simulink model "Model12"  (R2020a)
settings: Solver=ode15s  StartTime=0.0  StopTime=200  RelTol=1e-3
values from neighbouring files (symbols this model uses):
  Cf = 100000    [Model12_MATscript.m]
  Cr = 110000    [Model12_MATscript.m]
undefined symbols (not defined in the file or in its folder): a, a0, a1, a10, a11, a12, a13, a14, a15, a16, a17, a2, a3, a4, a5, a6, a7, a8, a9, alpha, Area, b, b1, b11, b12, b2, banking_indy, bankingON, C_fuel, camber, curveCenters, Cx, Cz, distanceThreshold, g, init_vel, init_x_pos, init_y_pos, init_yaw, IT, K_wear, l_f, l_r, longStraight, lookahead, m_fuel, mT, overlapThreshold, radius_second_lane, rho_0, rho_1, shortStraight, slipstreamON, trajec, turn, TyreContactAreaFront, TyreContactAreaRear, w1, w2
libraries: simulink x6
(part 2 of 2)

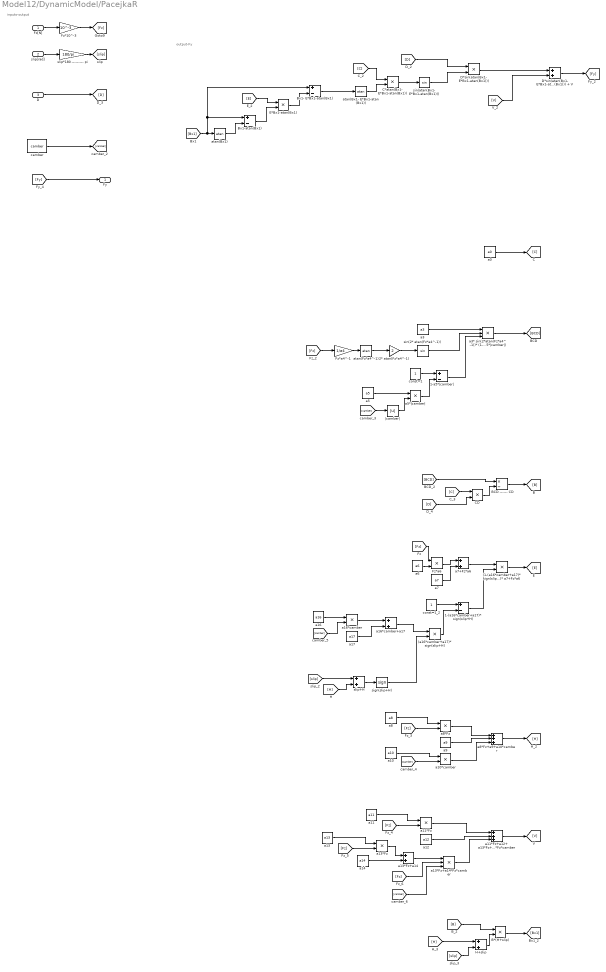
== system Model12/DynamicModel/PacejkaR ==
  note: inputs-output
  note: output-Fy
  Fz[N] : Inport  Unit=N
  slip[rad] : Inport  Port=2  Unit=rad
  D : Inport  Port=3
  (1-(a16*camber+a17)* sign(slip+H))* a7+Fz*a6 : Product
  (a16*camber+a17)* sign(slip+H) : Product
  1-(a16*camber+a17)* sign(slip+H) : Sum  Inputs=+-
  1-a5*|camber| : Sum  Inputs=+-
  2* atan(Fz*a4^-1) : Gain  Gain=2
  B*(H+slip) : Product
  BCD ------ CD : Product  Inputs=*/
  Bx1- E*Bx1-atan(Bx1) : Sum  Inputs=+-
  Bx1-atan(Bx1) : Sum  Inputs=+-
  C*atan(Bx1- E*Bx1-atan(Bx1)) : Product
  CD : Product
  D*sin(atan(Bx1- E*Bx1-atan(Bx1))) : Product
  D*sin(atan(Bx1- E*Bx1-atan(Bx1))) + V : Sum
  E*Bx1-atan(Bx1) : Product
  Fz*10^-3 : Gain  Gain=10^-3
  Fz*a4^-1 : Gain  Gain=1/a4
  Fz*a6 : Product
  H+slip : Sum
  a0 : Constant  Value=a0
  a10 : Constant  Value=a10
  a10*camber : Product
  a11 : Constant  Value=a11
  a11*Fz : Product
  a11*Fz+a12+ a13*Fz+a14*Fz*camber : Sum  Inputs=+++
  a12 : Constant  Value=a12
  a13 : Constant  Value=a13
  a13*Fz : Product
  a13*Fz+a14 : Sum
  a13*Fz+a14*Fz*camber : Product  Inputs=3
  a14 : Constant  Value=a14
  a16 : Constant  Value=a16
  a16*camber : Product
  a16*camber+a17 : Sum
  a17 : Constant  Value=a17
  a3 : Constant  Value=a3
  a3* sin(2*atan(Fz*a4^-1))* (1-a5*|camber|) : Product  Inputs=3
  a5 : Constant  Value=a5
  a5*|camber| : Product
  a6 : Constant  Value=a6
  a7 : Constant  Value=a7
  a7+Fz*a6 : Sum
  a8 : Constant  Value=a8
  a8*Fz : Product
  a8*Fz+a9+a10*camber : Sum  Inputs=+++
  a9 : Constant  Value=a9
  atan(Bx1) : Trigonometry  Operator=atan
  atan(Bx1- E*Bx1-atan(Bx1)) : Trigonometry  Operator=atan
  atan(Fz*a4^-1) : Trigonometry  Operator=atan
  camber : Constant  Value=camber
  const=1 : Constant
  const=1_2 : Constant
  sign(slip+H) : Signum  ZeroCross=off
  sin(2* atan(Fz*a4^-1)) : Trigonometry
  sin(atan(Bx1- E*Bx1-atan(Bx1))) : Trigonometry
  slip*180 --------- pi : Gain  Gain=180/pi
  slip+H : Sum
  |camber| : Abs
  Fy : Outport  Unit=N
  wires:
  C*atan(Bx1- E*Bx1-atan(Bx1))/1 -> sin(atan(Bx1- E*Bx1-atan(Bx1)))/1
  E*Bx1-atan(Bx1)/1 -> Bx1- E*Bx1-atan(Bx1)/2
  slip[rad]/1 -> slip*180 --------- pi/1
  1-a5*|camber|/1 -> a3* sin(2*atan(Fz*a4^-1))* (1-a5*|camber|)/3
  a10*camber/1 -> a8*Fz+a9+a10*camber/3
  |camber|/1 -> a5*|camber|/2
  a8/1 -> a8*Fz/1
  Fz*10^-3/1 -> [Fz]
  a0/1 -> [C]
  atan(Bx1- E*Bx1-atan(Bx1))/1 -> C*atan(Bx1- E*Bx1-atan(Bx1))/2
  [Fy] -> Fy/1
  Fz*a4^-1/1 -> atan(Fz*a4^-1)/1
  [B] -> B*(H+slip)/1
  [Fz] -> a8*Fz/2
  [Bx1] -> atan(Bx1)/1, Bx1-atan(Bx1)/1, Bx1- E*Bx1-atan(Bx1)/1
  [Fz] -> a13*Fz+a14*Fz*camber/2
  slip*180 --------- pi/1 -> [slip]
  2* atan(Fz*a4^-1)/1 -> sin(2* atan(Fz*a4^-1))/1
  [Fz] -> Fz*a6/1
  [slip] -> H+slip/2
  a11*Fz+a12+ a13*Fz+a14*Fz*camber/1 -> [V]
  a7+Fz*a6/1 -> (1-(a16*camber+a17)* sign(slip+H))* a7+Fz*a6/1
  [D] -> D*sin(atan(Bx1- E*Bx1-atan(Bx1)))/1
  a8*Fz+a9+a10*camber/1 -> [H]
  1-(a16*camber+a17)* sign(slip+H)/1 -> (1-(a16*camber+a17)* sign(slip+H))* a7+Fz*a6/2
  Bx1- E*Bx1-atan(Bx1)/1 -> atan(Bx1- E*Bx1-atan(Bx1))/1
  a3/1 -> a3* sin(2*atan(Fz*a4^-1))* (1-a5*|camber|)/1
  [camber] -> a16*camber/2
  [V] -> D*sin(atan(Bx1- E*Bx1-atan(Bx1))) + V/2
  [C] -> C*atan(Bx1- E*Bx1-atan(Bx1))/1
  B*(H+slip)/1 -> [Bx1]
  Fz[N]/1 -> Fz*10^-3/1
  camber/1 -> [camber]
  a11*Fz/1 -> a11*Fz+a12+ a13*Fz+a14*Fz*camber/1
  const=1/1 -> 1-a5*|camber|/1
  [Fz] -> a13*Fz/2
  a8*Fz/1 -> a8*Fz+a9+a10*camber/1
  [BCD] -> BCD ------ CD/1
  a14/1 -> a13*Fz+a14/2
  sin(atan(Bx1- E*Bx1-atan(Bx1)))/1 -> D*sin(atan(Bx1- E*Bx1-atan(Bx1)))/2
  sign(slip+H)/1 -> (a16*camber+a17)* sign(slip+H)/2
  a3* sin(2*atan(Fz*a4^-1))* (1-a5*|camber|)/1 -> [BCD]
  [camber] -> |camber|/1
  a13*Fz+a14/1 -> a13*Fz+a14*Fz*camber/1
  a9/1 -> a8*Fz+a9+a10*camber/2
  a16*camber/1 -> a16*camber+a17/1
  a12/1 -> a11*Fz+a12+ a13*Fz+a14*Fz*camber/2
  (1-(a16*camber+a17)* sign(slip+H))* a7+Fz*a6/1 -> [E]
  [Fz] -> Fz*a4^-1/1
  D*sin(atan(Bx1- E*Bx1-atan(Bx1))) + V/1 -> [Fy]
  BCD ------ CD/1 -> [B]
  a10/1 -> a10*camber/1
  [H] -> H+slip/1
  atan(Fz*a4^-1)/1 -> 2* atan(Fz*a4^-1)/1
  a16*camber+a17/1 -> (a16*camber+a17)* sign(slip+H)/1
  a11/1 -> a11*Fz/1
  a13*Fz/1 -> a13*Fz+a14/1
  a13*Fz+a14*Fz*camber/1 -> a11*Fz+a12+ a13*Fz+a14*Fz*camber/3
  a17/1 -> a16*camber+a17/2
  Fz*a6/1 -> a7+Fz*a6/1
  sin(2* atan(Fz*a4^-1))/1 -> a3* sin(2*atan(Fz*a4^-1))* (1-a5*|camber|)/2
  [Fz] -> a11*Fz/2
  [camber] -> a13*Fz+a14*Fz*camber/3
  Bx1-atan(Bx1)/1 -> E*Bx1-atan(Bx1)/2
  [C] -> CD/1
  [camber] -> a10*camber/2
  a6/1 -> Fz*a6/2
  [D] -> CD/2
  atan(Bx1)/1 -> Bx1-atan(Bx1)/2
  a13/1 -> a13*Fz/1
  (a16*camber+a17)* sign(slip+H)/1 -> 1-(a16*camber+a17)* sign(slip+H)/2
  D*sin(atan(Bx1- E*Bx1-atan(Bx1)))/1 -> D*sin(atan(Bx1- E*Bx1-atan(Bx1))) + V/1
  D/1 -> [D]
  H+slip/1 -> B*(H+slip)/2
  [E] -> E*Bx1-atan(Bx1)/1
  const=1_2/1 -> 1-(a16*camber+a17)* sign(slip+H)/1
  a7/1 -> a7+Fz*a6/2
  a16/1 -> a16*camber/1
  a5*|camber|/1 -> 1-a5*|camber|/2
  a5/1 -> a5*|camber|/1
  CD/1 -> BCD ------ CD/2
  [H] -> slip+H/2
  slip+H/1 -> sign(slip+H)/1
  [slip] -> slip+H/1

== matlab function Model12/Controller/Longitudinal_controller/v_ref ==
  data: egox input; egoy input; trajec input; ref output
function ref = vel_ref(egox, egoy, trajec)

% index = floor(mod(pos*10, max_pos) + 1);
% thresh1 = 60;
% thresh2 = 20;
% from = max(1, index - thresh1);
% to = min(max_pos, index + thresh2);
% 
% real_index = from;
% min_dist = pdist2([trajec(2,real_index),trajec(3,real_index)],[egox, egoy]);
% for i=from+1:to
%     new_dist = pdist2([trajec(2,i),trajec(3,i)],[egox, egoy]);
%     if new_dist < min_dist
%         min_dist = new_dist;
%         real_index = i;
%     end
% end
distArray = (egox - trajec(2,:)).^2 + (egoy - trajec(3,:)).^2;
[~, real_index] = min(distArray);
ref = trajec(5, real_index);

% function ref = vel_ref(egox, egoy, trajec, cur_vel)
% 
% thresh = 5;
% maxp = 10;
% index = find( (abs(trajec(2,:) - egox) < thresh) & (abs(trajec(3,:) - egoy) < thresh), maxp);
% 
% if (isempty(index))
%     ref = cur_vel;
% else
%     
%     size_index = size(index, 2);
% 
%     real_index = index(1,1);
%     min_dist = pdist2([trajec(2,real_index),trajec(3,real_index)],[egox, egoy]);
% 
%     for i=2:size_index
%         new_dist = pdist2([trajec(2,index(1,i)),trajec(3,index(1,i))],[egox, egoy]);
%         if new_dist < min_dist
%             min_dist = new_dist;
%             real_index = index(1,i);
%         end
%     end
%     
%     ref = trajec(5, real_index);
% end

== matlab function Model12/DynamicModel/Banking ==
  data: x input; res output; y input; curveCenters input; longStraight input; shortStraight input; curve input; bankingON input; banking_indy input
function res = calculateBanking(x, y, curveCenters, ...
    longStraight, shortStraight, curve, ...
    bankingON, banking_indy)

% coder.extrinsic('evalin')
% coder.extrinsic('fitresult')
% fun = evalin('base','fitresult');

init_x = -271.4;
totL = 4023.4;
initD = pdist2([init_x, 0], [curveCenters(1,1),0]);

R = curve * 2 / pi;


if (bankingON < 1)
    res = 0;
else
    % long straight 1
    if y < curveCenters(1,2) && x >= curveCenters(4,1) && x <= curveCenters(1,1)
        d = pdist2([x, 0],[init_x, 0]);
        l = (totL - d)*(x < init_x) + ...
            (d)*(x >= init_x);
    % long straight 2
    elseif y > curveCenters(2,2) && x >= curveCenters(4,1) && x <= curveCenters(1,1)
        d = pdist2([x, 0],[curveCenters(2,1),0]);
        l = d + initD + shortStraight + 2*curve;
    % short straigt 1
    elseif x > 0 && y >= curveCenters(1,2) && y <= curveCenters(2,2)
        d = pdist2([y, 0],[curveCenters(1,2),0]);
        l = d + initD + curve;
    % short straigt 2
    elseif x < 0 && y >= curveCenters(1,2) && y <= curveCenters(2,2)
        d = pdist2([y, 0],[curveCenters(3,2),0]);
        l = d + initD + longStraight + shortStraight + 3*curve;
    % curve 1
    elseif x > curveCenters(1,1) && y < curveCenters(1,2)
        ang = asin((x - curveCenters(1,1))/pdist2([x,y],curveCenters(1,:)));
        l = ang * R + initD;
    % curve 2
    elseif x > curveCenters(2,1) && y > curveCenters(2,2)
        ang = asin((y - curveCenters(2,2))/pdist2([x,y],curveCenters(2,:)));
        l = ang * R + initD + curve + shortStraight;
    % curve 3
    elseif x < curveCenters(3,1) && y > curveCenters(3,2)
        ang = asin((-x + curveCenters(3,1))/pdist2([x,y],curveCenters(3,:)));
        l = ang * R + initD + curve*2 + shortStraight + longStraight;
    % curve 4
    elseif x < curveCenters(4,1) && y < curveCenters(4,2)
        ang = asin((-y + curveCenters(4,2))/pdist2([x,y],curveCenters(4,:)));
        l = ang * R + initD + curve*3 + shortStraight*2 + longStraight;
    % default else
    else 
        l = 0;
    end
    
    %res = fun(l);
    res = banking_indy(ceil(l*10),1);
    %res = 0;
end

% function res = calculateBanking(x, y, curveCenters, ...
%     bankingThresholdLong, bankingThresholdShort, bankingAngle, midY, ...
%     bankingON)
% if (bankingON < 1)
%     res = 0;
% else
%     if(y < curveCenters(1,2) || y > curveCenters(2,2)) 
%        if(abs(x) < curveCenters(1,1) - bankingThresholdLong)
%            res = 0;
%        elseif (abs(x) > curveCenters(1,1))
%            res = bankingAngle;
%        else
%            res = bankingAngle*( 1 - ((abs(x) -  curveCenters(1,1))/(-bankingThresholdLong)) );
%        end
%     else
%         if (abs(y-midY) < curveCenters(2,2) - bankingThresholdShort - midY)
%             res = 0;
%         else
%             res = bankingAngle*( 1 - ((abs(y-midY) -  curveCenters(2,2) + midY)/(-bankingThresholdShort)) );
%         end
%     end
% end

== matlab function Model12/Controller/Lateral_controller/periodic ==
  data: yaw input; periodicYaw output
function periodicYaw = periodic(yaw)

periodicYaw = abs(yaw) - (2*pi * floor(abs(yaw)/(2*pi)));

== matlab function Model12/DynamicModel/WindEffect ==
  data: rho_0 input; aerodynamic_coeff output; rho_1 input; ego_x input; ego_y input; opp_x input; opp_y input; distanceThreshold input; overlapThreshold input; alpha input; curveCenters input; slipstreamON input
function aerodynamic_coeff = windEffect(rho_0, rho_1, ego_x, ego_y, ... 
    opp_x, opp_y, distanceThreshold, overlapThreshold, alpha, curveCenters, ...
    slipstreamON)

if(slipstreamON < 1)
    aerodynamic_coeff = rho_0;
else
    %give in output rho_0 if too distant from other vehicle
    %rho_1 otherwise
    distanceThresholdCurve =  alpha * distanceThreshold;
    overlapThresholdCurve =  alpha * overlapThreshold;

    if  ego_x > curveCenters(1,1) && ego_y < curveCenters(1,2) %check if in the first curve
        ego_radius = sqrt((ego_x - curveCenters(1,1))^2 + (ego_y - curveCenters(1,2))^2);
        opp_radius = sqrt((opp_x - curveCenters(1,1))^2 + (opp_y - curveCenters(1,2))^2);
        if abs(ego_radius - opp_radius) < overlapThresholdCurve && ...
                sqrt((ego_x - opp_x)^2 + (ego_y - opp_y)^2) < distanceThresholdCurve && ...
                ego_y < opp_y
            aerodynamic_coeff = rho_1;
        else
           aerodynamic_coeff = rho_0;
        end
    elseif ego_x > curveCenters(2,1) && ego_y > curveCenters(2,2) %check if in the second curve
        ego_radius = sqrt((ego_x - curveCenters(2,1))^2 + (ego_y - curveCenters(2,2))^2);
        opp_radius = sqrt((opp_x - curveCenters(2,1))^2 + (opp_y - curveCenters(2,2))^2);
        if abs(ego_radius - opp_radius) < overlapThresholdCurve && ...
                sqrt((ego_x - opp_x)^2 + (ego_y - opp_y)^2) < distanceThresholdCurve && ...
                ego_x > opp_x
            aerodynamic_coeff = rho_1;
        else
           aerodynamic_coeff = rho_0;
        end
    elseif ego_x < curveCenters(3,1) && ego_y > curveCenters(3,2) %check if in the third curve
        ego_radius = sqrt((ego_x - curveCenters(3,1))^2 + (ego_y - curveCenters(3,2))^2);
        opp_radius = sqrt((opp_x - curveCenters(3,1))^2 + (opp_y - curveCenters(3,2))^2);
        if abs(ego_radius - opp_radius) < overlapThresholdCurve && ...
                sqrt((ego_x - opp_x)^2 + (ego_y - opp_y)^2) < distanceThresholdCurve && ...
                ego_y > opp_y
            aerodynamic_coeff = rho_1;
        else
           aerodynamic_coeff = rho_0;
        end
    elseif ego_x < curveCenters(4,1) && ego_y < curveCenters(4,2) %check if in the fourth curve
        ego_radius = sqrt((ego_x - curveCenters(4,1))^2 + (ego_y - curveCenters(4,2))^2);
        opp_radius = sqrt((opp_x - curveCenters(4,1))^2 + (opp_y - curveCenters(4,2))^2);
        if abs(ego_radius - opp_radius) < overlapThresholdCurve && ...
                sqrt((ego_x - opp_x)^2 + (ego_y - opp_y)^2) < distanceThresholdCurve && ...
                ego_x < opp_x
            aerodynamic_coeff = rho_1;
        else
           aerodynamic_coeff = rho_0;
        end
    else
        %check for which straights
        if ego_y < curveCenters(1,2) && ego_x >= curveCenters(4,1) && ego_x <= curveCenters(1,1)
           %first long straight
           if abs(ego_y - opp_y) < overlapThreshold && ...
                   abs(opp_x - ego_x) < distanceThreshold && ...
                   ego_x < opp_x
               aerodynamic_coeff = rho_1;
           else
               aerodynamic_coeff = rho_0;
           end

        elseif ego_y > curveCenters(2,2) && ego_x >= curveCenters(3,1) && ego_x <= curveCenters(2,1)
           %second long straight
           if abs(ego_y - opp_y) < overlapThreshold && ...
                   abs(opp_x - ego_x) < distanceThreshold && ...
                   ego_x > opp_x
               aerodynamic_coeff = rho_1;
           else
               aerodynamic_coeff = rho_0;
           end

        elseif ego_x > curveCenters(1,1) && ego_y >= curveCenters(1,2) && ego_y <= curveCenters(2,2)
           %first short straight
           if abs(ego_x - opp_x) < overlapThreshold && ...
                   abs(opp_y - ego_y) < distanceThreshold && ...
                   ego_y < opp_y
               aerodynamic_coeff = rho_1;
           else
               aerodynamic_coeff = rho_0;
           end

        elseif ego_x < curveCenters(3,1) && ego_y >= curveCenters(4,2) && ego_y <= curveCenters(3,2)
           %second short straight
           if abs(ego_x - opp_x) < overlapThreshold && ...
                   abs(opp_y - ego_y) < distanceThreshold && ...
                   ego_y > opp_y
               aerodynamic_coeff = rho_1;
           else
               aerodynamic_coeff = rho_0;
           end

        else
            aerodynamic_coeff = rho_0;
        end
    end
end

== matlab function Model12/Controller/Lateral_controller/lateral error ==
  data: egox input; egoy input; trajec input; error_la output; curv output; cur_yaw input; index output; lookAhead input; curveCenters input; e output; radiusTrajec input
function [error_la,curv,index, e] = lateral_error(egox, egoy, trajec, cur_yaw, lookAhead, curveCenters, radiusTrajec)

distArrayEgo = (egox - trajec(2,:)).^2 + (egoy - trajec(3,:)).^2;
[min_dist_ego, ~] = min(distArrayEgo);

e = sqrt(min_dist_ego);


newEgox = egox + lookAhead*cos(cur_yaw);
newEgoy = egoy + lookAhead*sin(cur_yaw);

distArray = (newEgox - trajec(2,:)).^2 + (newEgoy - trajec(3,:)).^2;
[min_dist, real_index] = min(distArray);

min_dist = sqrt(min_dist);

index = real_index; %output

v1 = [newEgox - egox, newEgoy - egoy, 0];
v2 = [trajec(2, real_index) - newEgox, trajec(3, real_index) - newEgoy, 0];
C = cross(v1, v2);

if sign(C(3)) == 1
    error_la = -min_dist;
elseif sign(C(3)) == -1
    error_la = min_dist;
else
    error_la = 0;
end


% long straight 1
if egoy < curveCenters(1,2) && egox >= curveCenters(4,1) && egox <= curveCenters(1,1)
    curv = 0;
elseif egoy > curveCenters(2,2) && egox >= curveCenters(4,1) && egox <= curveCenters(1,1)
    curv = 0;
% short straigt 1
elseif egox > 0 && egoy >= curveCenters(1,2) && egoy <= curveCenters(2,2)
    curv = 0;
% short straigt 2
elseif egox < 0 && egoy >= curveCenters(1,2) && egoy <= curveCenters(2,2)
    curv = 0;
% curve 1
elseif egox > curveCenters(1,1) && egoy < curveCenters(1,2)
    curv = 1/radiusTrajec;
% curve 2
elseif egox > curveCenters(2,1) && egoy > curveCenters(2,2)
    curv = 1/radiusTrajec;
% curve 3
elseif egox < curveCenters(3,1) && egoy > curveCenters(3,2)
    curv = 1/radiusTrajec;
% curve 4
elseif egox < curveCenters(4,1) && egoy < curveCenters(4,2)
    curv = 1/radiusTrajec;
% default else
else
    curv = 0;
end



% % long straight 1
% if newEgoy < curveCenters(1,2) && newEgox >= curveCenters(4,1) && newEgox <= curveCenters(1,1)
%     curv = 0;
% % elseif newEgoy < curveCenters(1,2) && newEgox >= curveCenters(4,1) + 100 && newEgox <= curveCenters(1,1)
% %     trajR = pdist2([trajec(2, real_index),trajec(3, real_index)],curveCenters(1,:));
% %     curv = 1/trajR;
% %     curv = curv * (abs(newEgox) - curveCenters(1,1) + 100) / 100;
% % long straight 2
% elseif newEgoy > curveCenters(2,2) && newEgox >= curveCenters(4,1) && newEgox <= curveCenters(1,1)
%     curv = 0;
% % short straigt 1
% elseif newEgox > 0 && newEgoy >= curveCenters(1,2) && newEgoy <= curveCenters(2,2)
%     curv = 0;
% % short straigt 2
% elseif newEgox < 0 && newEgoy >= curveCenters(1,2) && newEgoy <= curveCenters(2,2)
%     curv = 0;
% % curve 1
% elseif newEgox > curveCenters(1,1) && newEgoy < curveCenters(1,2)
%     trajR = pdist2([trajec(2, real_index),trajec(3, real_index)],curveCenters(1,:));
%     curv = 1/trajR;
% % curve 2
% elseif newEgox > curveCenters(2,1) && newEgoy > curveCenters(2,2)
%     trajR = pdist2([trajec(2, real_index),trajec(3, real_index)],curveCenters(2,:));
%     curv = 1/trajR;
% % curve 3
% elseif newEgox < curveCenters(3,1) && newEgoy > curveCenters(3,2)
%     trajR = pdist2([trajec(2, real_index),trajec(3, real_index)],curveCenters(3,:));
%     curv = 1/trajR;
% % curve 4
% elseif newEgox < curveCenters(4,1) && newEgoy < curveCenters(4,2)
%     trajR = pdist2([trajec(2, real_index),trajec(3, real_index)],curveCenters(4,:));
%     curv = 1/trajR;
% % default else
% else
%     curv = 0;
% end
